simulink model "mdl_positionLoop_2"  (R2022b)
settings: Solver=VariableStepAuto  StartTime=0.0  StopTime=2  RelTol=1e-3
values from neighbouring files (symbols this model uses):
  J = 0.00016    [m2_5_1.m]    (also in m2_5_2.m)
undefined symbols (not defined in the file or in its folder): sigbuilder_block
settings Model: Creator=jack  LastModifiedBy=jackyeh

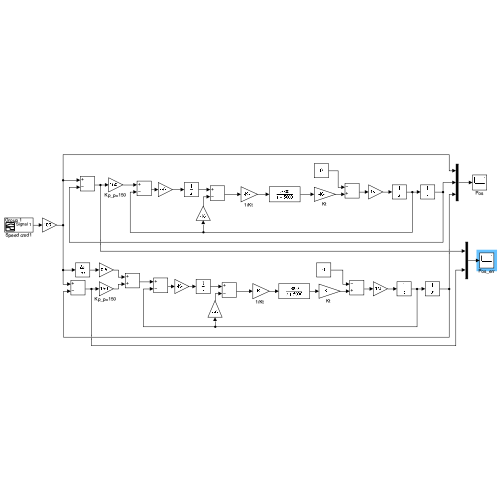
[thumbnail: Simulink's stored preview of the top-level diagram]
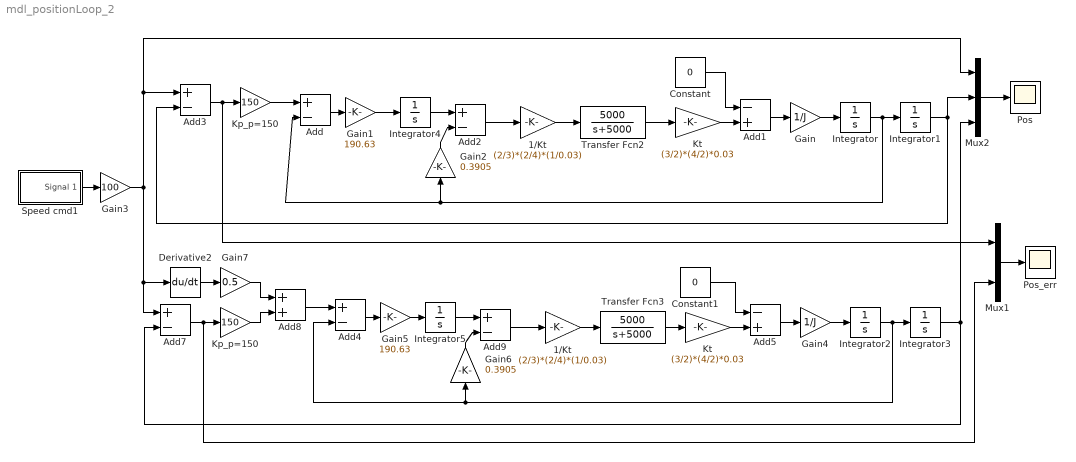
== system mdl_positionLoop_2 ==
  "1/Kt " : Gain  Gain=(2/3)*(2/4)*(1/0.03)
  "1/Kt  " : Gain  Gain=(2/3)*(2/4)*(1/0.03)
  Add{,2..4,7,9} (6 alike) : Sum  Inputs=+-
  Add1 : Sum  Inputs=-+
  Add5 : Sum  Inputs=-+
  Add8 : Sum
  Constant : Constant  Value=0
  Constant1 : Constant  Value=0
  Derivative2 : Derivative
  Gain : Gain  Gain=1/J
  Gain1 : Gain  Gain=190.63
  Gain2 : Gain  Gain=0.3905
  Gain3 : Gain  Gain=100
  Gain4 : Gain  Gain=1/J
  Gain5 : Gain  Gain=190.63
  Gain6 : Gain  Gain=0.3905
  Gain7 : Gain  Gain=0.5
  Integrator{,1..5} (6 alike) : Integrator
  Kp_p=150 : Gain  Gain=150
  "Kp_p=150 " : Gain  Gain=150
  "Kt " : Gain  Gain=(3/2)*(4/2)*0.03
  "Kt  " : Gain  Gain=(3/2)*(4/2)*0.03
  Mux1 : Mux  Inputs=2
  Mux2 : Mux  Inputs=3
  Pos : Scope
  Pos_err : Scope
  Speed cmd1 : Subsystem  Tag=STV Subsys  LoadFcn=sigbuilder_block('load');  StartFcn=sigbuilder_block('start');  StopFcn=sigbuilder_block('stop');  ClipboardFcn=sigbuilder_block('clipboard');  mask(Sigbuilder block){tuvar=[0:10]}
      mask help: Simulink:masks:SigbuilderBlock_MD
      mask init:
      | if ~strcmp(get_param(bdroot(gcbh),'SimulationStatus'),'stopped') tuvar = sigbuilder_block('maskInit'); end
      settings: CopyFcn=sigbuilder_block('copy');  DeleteFcn=sigbuilder_block('delete');  ModelCloseFcn=sigbuilder_block('modelClose');  PreSaveFcn=sigbuilder_block('preSave');  PauseFcn=sigbuilder_block('pause');  ContinueFcn=sigbuilder_block('continue');  NameChangeFcn=sigbuilder_block('namechange');  OpenFcn=sigbuilder_block('open',[437.6 199.2 550.4 400 ]);  CloseFcn=sigbuilder_block('close');
      mask Display: plot(0, 0, 100, 100,[2, 2, 32, 32, 2], [68, 8, 8, 68, 68],[32, 2], [38, 38], [32, 19, 2],[53, 60, 44], [32, 17, 17, 2],[16, 16, 31, 31]);txt = getActiveGroup(gcbh);text(2, 100, txt,'verticalAlignment', 'top');
  Transfer Fcn2 : TransferFcn  Numerator=[5000]  Denominator=[1 5000]
  Transfer Fcn3 : TransferFcn  Numerator=[5000]  Denominator=[1 5000]
  wires:
  Gain/1 -> Integrator/1
  Integrator/1 -> Integrator1/1, Gain2/1, Add/2
  Constant/1 -> Add1/1
  Add1/1 -> Gain/1
  Add2/1 -> "1/Kt "/1
  Mux2/1 -> Pos/1
  "1/Kt "/1 -> Transfer Fcn2/1
  "Kt "/1 -> Add1/2
  Speed cmd1/1(Signal 1) -> Gain3/1
  Transfer Fcn2/1 -> "Kt "/1
  Add3/1 -> Mux1/1, Kp_p=150/1
  Gain3/1 -> Add3/1, Mux2/1, Derivative2/1, Add7/1
  Kp_p=150/1 -> Add/1
  Integrator1/1 -> Mux2/2, Add3/2
  Integrator3/1 -> Mux2/3, Add7/2
  Add7/1 -> Mux1/2, "Kp_p=150 "/1
  Transfer Fcn3/1 -> "Kt  "/1
  "Kt  "/1 -> Add5/2
  "1/Kt  "/1 -> Transfer Fcn3/1
  Add5/1 -> Gain4/1
  Constant1/1 -> Add5/1
  Integrator2/1 -> Add4/2, Gain6/1, Integrator3/1
  Gain4/1 -> Integrator2/1
  "Kp_p=150 "/1 -> Add8/2
  Add8/1 -> Add4/1
  Mux1/1 -> Pos_err/1
  Gain7/1 -> Add8/1
  Derivative2/1 -> Gain7/1
  Add/1 -> Gain1/1
  Gain1/1 -> Integrator4/1
  Integrator4/1 -> Add2/1
  Gain2/1 -> Add2/2
  Gain6/1 -> Add9/2
  Integrator5/1 -> Add9/1
  Gain5/1 -> Integrator5/1
  Add9/1 -> "1/Kt  "/1
  Add4/1 -> Gain5/1

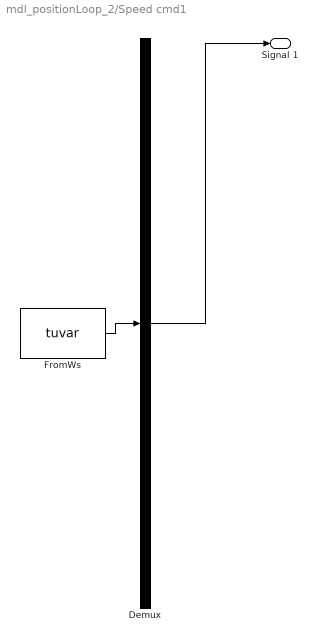
== system mdl_positionLoop_2/Speed cmd1 ==
  Demux : Demux  Tag=STV Demux  Outputs=1
      settings: DisplayOption=none
  FromWs : FromWorkspace  Tag=STV FromWs  VariableName=tuvar
      SigBuilderData=|
      | common.afterFinalStr = 'Extrapolate'
      | common.sampleTime = 0
      | dataSet.timeRange = [0 10]
      | dataSet.name = 'Group 1'
      | sbobj.Groups.Name = 'Group 1'
      | sbobj.Groups.Signals.Name = 'Signal 1'
      | sbobj.Groups.Signals.XData = [0 0.01 0.5 1 1.01 10]
      | sbobj.Groups.Signals.YData = [0.005 1 1 1 0 0]
  Signal 1 : Outport  Tag=STV Outport
  wires:
  Demux/1 -> Signal 1/1
  FromWs/1 -> Demux/1
